simulink model "momentumBasedFlying"  (Simulink 10.3)
settings: Solver=FixedStepAuto  StartTime=0.0  StopTime=Config.simulationTime  FixedStep=Config.tStep  RelTol=1e-3
InitFcn:
  | cd(fileparts(which(bdroot)));
  | initMomentumBasedFlying;
StopFcn:
  | cd(fileparts(which(bdroot)));
  | stopMomentumBasedFlying;
undefined symbols (not defined in the file or in its folder): biasVectorConstraint_feet, Config, confVisualizer, ConstraintMatrix_feet, DiscIntNeverNeededParam, jets_config
libraries: WBToolboxLibrary x95, momentum_flight_control_sublib x2
(part 4 of 5)

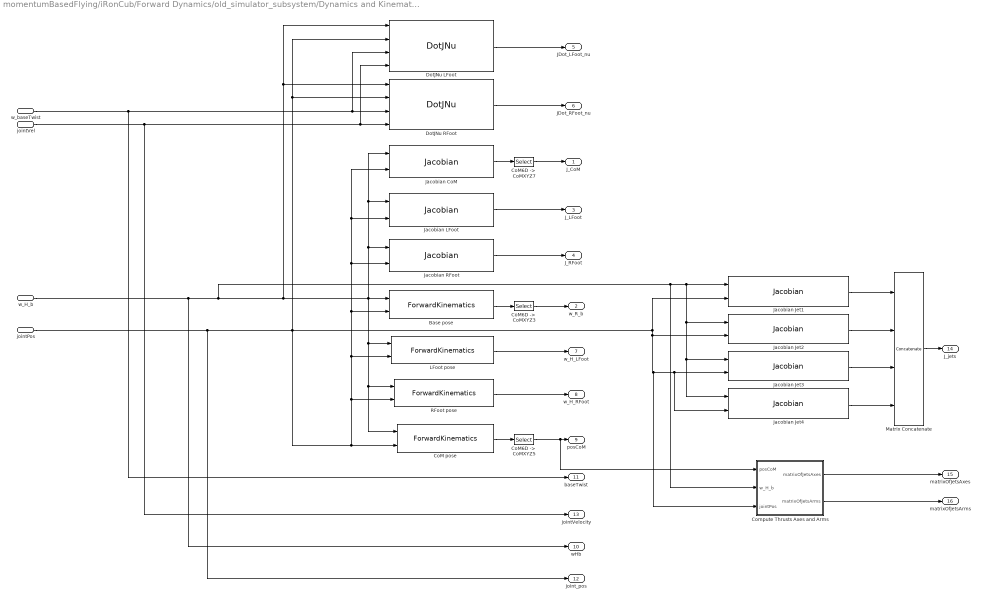
== system momentumBasedFlying/iRonCub/Forward Dynamics/old_simulator_subsystem/Dynamics and Kinematics/Kinematic Quantities ==
  w_H_b : Inport
  w_baseTwist : Inport  Port=2
  jointPos : Inport  Port=3
  jointVel : Inport  Port=4
  Base pose : WBToolboxLibrary/Model/Kinematics/ForwardKinematics  frameName=Frames.BASE_LINK
      settings: SourceProductName=WholeBodyToolbox
  CoM pose : WBToolboxLibrary/Model/Kinematics/ForwardKinematics  frameName=Frames.COM_FRAME
      settings: SourceProductName=WholeBodyToolbox
  "CoM6D ->  CoMXYZ3" : Selector  NumberOfDimensions=2  InputPortWidth=7  IndexOptions=Index vector (dialog),Index vector (dialog)  Indices=[1 2 3],[1 2 3]  OutputSizes=1,1
  "CoM6D ->  CoMXYZ5" : Selector  NumberOfDimensions=2  InputPortWidth=7  IndexOptions=Index vector (dialog),Index vector (dialog)  Indices=[1 2 3],[4]  OutputSizes=1,1
  "CoM6D ->  CoMXYZ7" : Selector  NumberOfDimensions=2  InputPortWidth=7  IndexOptions=Index vector (dialog),Index vector (dialog)  Indices=[1 2 3],[1:6+Config.N_DOF]  OutputSizes=1,1
  Compute Thrusts Axes and Arms : Subsystem
  DotJNu LFoot : WBToolboxLibrary/Model/Jacobians/DotJNu  frameName=Frames.LFOOT_FRAME
      settings: SourceProductName=WholeBodyToolbox
  DotJNu RFoot : WBToolboxLibrary/Model/Jacobians/DotJNu  frameName=Frames.RFOOT_FRAME
      settings: SourceProductName=WholeBodyToolbox
  Jacobian CoM : WBToolboxLibrary/Model/Jacobians/Jacobian  frameName=Frames.COM_FRAME
      settings: SourceProductName=WholeBodyToolbox
  Jacobian Jet1 : WBToolboxLibrary/Model/Jacobians/Jacobian  frameName=Frames.JET1_FRAME
      settings: SourceProductName=WholeBodyToolbox
  Jacobian Jet2 : WBToolboxLibrary/Model/Jacobians/Jacobian  frameName=Frames.JET2_FRAME
      settings: SourceProductName=WholeBodyToolbox
  Jacobian Jet3 : WBToolboxLibrary/Model/Jacobians/Jacobian  frameName=Frames.JET3_FRAME
      settings: SourceProductName=WholeBodyToolbox
  Jacobian Jet4 : WBToolboxLibrary/Model/Jacobians/Jacobian  frameName=Frames.JET4_FRAME
      settings: SourceProductName=WholeBodyToolbox
  Jacobian LFoot : WBToolboxLibrary/Model/Jacobians/Jacobian  frameName=Frames.LFOOT_FRAME
      settings: SourceProductName=WholeBodyToolbox
  Jacobian RFoot : WBToolboxLibrary/Model/Jacobians/Jacobian  frameName=Frames.RFOOT_FRAME
      settings: SourceProductName=WholeBodyToolbox
  LFoot pose : WBToolboxLibrary/Model/Kinematics/ForwardKinematics  frameName=Frames.LFOOT_FRAME
      settings: SourceProductName=WholeBodyToolbox
  Matrix Concatenate : Concatenate  NumInputs=4  Mode=Multidimensional array
  RFoot pose : WBToolboxLibrary/Model/Kinematics/ForwardKinematics  frameName=Frames.RFOOT_FRAME
      settings: SourceProductName=WholeBodyToolbox
  J_CoM : Outport  VectorParamsAs1DForOutWhenUnconnected=off
  w_R_b : Outport  Port=2  VectorParamsAs1DForOutWhenUnconnected=off
  J_LFoot : Outport  Port=3  VectorParamsAs1DForOutWhenUnconnected=off
  J_RFoot : Outport  Port=4  VectorParamsAs1DForOutWhenUnconnected=off
  JDot_LFoot_nu : Outport  Port=5  VectorParamsAs1DForOutWhenUnconnected=off
  JDot_RFoot_nu : Outport  Port=6  VectorParamsAs1DForOutWhenUnconnected=off
  w_H_LFoot : Outport  Port=7  VectorParamsAs1DForOutWhenUnconnected=off
  w_H_RFoot : Outport  Port=8  VectorParamsAs1DForOutWhenUnconnected=off
  posCoM : Outport  Port=9  VectorParamsAs1DForOutWhenUnconnected=off
  wHb : Outport  Port=10
  baseTwist : Outport  Port=11
  joint_pos : Outport  Port=12
  jointVelocity : Outport  Port=13
  J_jets : Outport  Port=14  VectorParamsAs1DForOutWhenUnconnected=off
  matrixOfJetsAxes : Outport  Port=15  VectorParamsAs1DForOutWhenUnconnected=off
  matrixOfJetsArms : Outport  Port=16  VectorParamsAs1DForOutWhenUnconnected=off
  wires:
  CoM pose/1 -> "CoM6D ->  CoMXYZ5"/1
  "CoM6D ->  CoMXYZ3"/1 -> w_R_b/1
  Jacobian CoM/1 -> "CoM6D ->  CoMXYZ7"/1
  Jacobian RFoot/1 -> J_RFoot/1
  Jacobian LFoot/1 -> J_LFoot/1
  DotJNu RFoot/1 -> JDot_RFoot_nu/1
  DotJNu LFoot/1 -> JDot_LFoot_nu/1
  jointVel/1 -> jointVelocity/1, DotJNu RFoot/4, DotJNu LFoot/4
  w_baseTwist/1 -> baseTwist/1, DotJNu LFoot/3, DotJNu RFoot/3
  RFoot pose/1 -> w_H_RFoot/1
  LFoot pose/1 -> w_H_LFoot/1
  Base pose/1 -> "CoM6D ->  CoMXYZ3"/1
  "CoM6D ->  CoMXYZ7"/1 -> J_CoM/1
  Compute Thrusts Axes and Arms/1(matrixOfJetsAxes) -> matrixOfJetsAxes/1
  Compute Thrusts Axes and Arms/2(matrixOfJetsArms) -> matrixOfJetsArms/1
  w_H_b/1 -> Compute Thrusts Axes and Arms/2(w_H_b), Jacobian Jet4/1, Jacobian Jet3/1, Jacobian Jet2/1, Jacobian Jet1/1, DotJNu LFoot/1, DotJNu RFoot/1, Jacobian LFoot/1, Jacobian CoM/1, Jacobian RFoot/1, CoM pose/1, RFoot pose/1, LFoot pose/1, Base pose/1, wHb/1
  Matrix Concatenate/1 -> J_jets/1
  Jacobian Jet3/1 -> Matrix Concatenate/3
  jointPos/1 -> Jacobian Jet4/2, Jacobian Jet3/2, Compute Thrusts Axes and Arms/3(jointPos), Jacobian Jet2/2, Jacobian Jet1/2, LFoot pose/2, Jacobian RFoot/2, Jacobian LFoot/2, Jacobian CoM/2, Base pose/2, RFoot pose/2, CoM pose/2, DotJNu RFoot/2, DotJNu LFoot/2, joint_pos/1
  Jacobian Jet4/1 -> Matrix Concatenate/4
  Jacobian Jet1/1 -> Matrix Concatenate/1
  Jacobian Jet2/1 -> Matrix Concatenate/2
  "CoM6D ->  CoMXYZ5"/1 -> Compute Thrusts Axes and Arms/1(posCoM), posCoM/1

== system momentumBasedFlying/FLYING CONTROLLER (CORE) V2.5/Dynamics and Kinematics/Dynamic Quantities/Momentum and CentroidalMomentum Matrix/CentroidalMomentum Matrix iCub 23/25 DoFs/CMM_base ==
  w_H_b : Inport
  jointPos : Inport  Port=2
  CentroidalMomentum{21..25,31} (6 alike) : WBToolboxLibrary/Model/Dynamics/CentroidalMomentum
      settings: SourceProductName=WholeBodyToolbox
  Constant : Constant  Value=[1,0,0,0,0,0]
  Constant1 : Constant  Value=[0,1,0,0,0,0]
  Constant2 : Constant  Value=zeros(Config.N_DOF,1)
  Constant3 : Constant  Value=[0,0,0,1,0,0]
  Constant37 : Constant  Value=[0,0,1,0,0,0]
  Constant4 : Constant  Value=[0,0,0,0,1,0]
  Constant6 : Constant  Value=[0,0,0,0,0,1]
  Matrix Concatenate : Concatenate  NumInputs=6  Mode=Multidimensional array  ConcatenateDimension=2
  CMM_base : Outport  VectorParamsAs1DForOutWhenUnconnected=off
  wires:
  w_H_b/1 -> CentroidalMomentum31/1, CentroidalMomentum25/1, CentroidalMomentum24/1, CentroidalMomentum23/1, CentroidalMomentum22/1, CentroidalMomentum21/1
  jointPos/1 -> CentroidalMomentum31/2, CentroidalMomentum25/2, CentroidalMomentum24/2, CentroidalMomentum23/2, CentroidalMomentum22/2, CentroidalMomentum21/2
  CentroidalMomentum25/1 -> Matrix Concatenate/5
  Matrix Concatenate/1 -> CMM_base/1
  CentroidalMomentum23/1 -> Matrix Concatenate/3
  CentroidalMomentum24/1 -> Matrix Concatenate/4
  CentroidalMomentum31/1 -> Matrix Concatenate/6
  Constant6/1 -> CentroidalMomentum31/3
  Constant/1 -> CentroidalMomentum21/3
  Constant1/1 -> CentroidalMomentum22/3
  Constant37/1 -> CentroidalMomentum23/3
  Constant2/1 -> CentroidalMomentum21/4, CentroidalMomentum31/4, CentroidalMomentum25/4, CentroidalMomentum24/4, CentroidalMomentum23/4, CentroidalMomentum22/4
  Constant4/1 -> CentroidalMomentum25/3
  Constant3/1 -> CentroidalMomentum24/3
  CentroidalMomentum22/1 -> Matrix Concatenate/2
  CentroidalMomentum21/1 -> Matrix Concatenate/1

== system momentumBasedFlying/FLYING CONTROLLER (CORE) V2.5/Dynamics and Kinematics/Dynamic Quantities/Momentum and CentroidalMomentum Matrix/CentroidalMomentum Matrix iCub 23/25 DoFs/CMM_joints ==
  w_H_b : Inport
  jointPos : Inport  Port=2
  SelMatrix : Inport  Port=3
  CMM Joints Group 1 : Subsystem
  CMM Joints Group 2 : Subsystem
  CMM Joints Group 3 : Subsystem
  CMM Joints Group 4 : Subsystem
  CMM Joints Group 5 : Subsystem
  Matrix Concatenate6 : Concatenate  NumInputs=4  Mode=Multidimensional array  ConcatenateDimension=2
  CMM_joints_from_1_to_20 : Outport  VectorParamsAs1DForOutWhenUnconnected=off
  CMM_group5_25DoFs : Outport  Port=2  VectorParamsAs1DForOutWhenUnconnected=off
  CMM_group5_23DoFs : Outport  Port=3  VectorParamsAs1DForOutWhenUnconnected=off
  wires:
  Matrix Concatenate6/1 -> CMM_joints_from_1_to_20/1
  w_H_b/1 -> CMM Joints Group 1/1(w_H_b), CMM Joints Group 2/1(w_H_b), CMM Joints Group 3/1(w_H_b), CMM Joints Group 4/1(w_H_b), CMM Joints Group 5/1(w_H_b)
  jointPos/1 -> CMM Joints Group 2/2(jointPos), CMM Joints Group 1/2(jointPos), CMM Joints Group 3/2(jointPos), CMM Joints Group 4/2(jointPos), CMM Joints Group 5/2(jointPos)
  SelMatrix/1 -> CMM Joints Group 3/3(SelMatrix), CMM Joints Group 2/3(SelMatrix), CMM Joints Group 1/3(SelMatrix), CMM Joints Group 4/3(SelMatrix), CMM Joints Group 5/3(SelMatrix)
  CMM Joints Group 1/1(CMM_group1) -> Matrix Concatenate6/1
  CMM Joints Group 2/1(CMM_group2) -> Matrix Concatenate6/2
  CMM Joints Group 3/1(CMM_group3) -> Matrix Concatenate6/3
  CMM Joints Group 4/1(CMM_group4) -> Matrix Concatenate6/4
  CMM Joints Group 5/1(CMM_group5_25DoFs) -> CMM_group5_25DoFs/1
  CMM Joints Group 5/2(CMM_group5_23DoFs) -> CMM_group5_23DoFs/1

== system momentumBasedFlying/FLYING CONTROLLER (CORE) V2.5/Dynamics and Kinematics/Dynamic Quantities/Momentum and CentroidalMomentum Matrix/CentroidalMomentum Matrix iCub 23/25 DoFs/Combine CMM ==
  CMM_base : Inport
  CMM_joints_1_20 : Inport  Port=2
  CMM_group5_25DoFs : Inport  Port=3
  CMM_group5_23DoFs : Inport  Port=4
  Matrix Concatenate1 : Concatenate  Mode=Multidimensional array  ConcatenateDimension=2
  Matrix Concatenate2 : Concatenate  Mode=Multidimensional array  ConcatenateDimension=2
  Matrix Concatenate6 : Concatenate  Mode=Multidimensional array  ConcatenateDimension=2
  CMM_25DoFs : Outport  VectorParamsAs1DForOutWhenUnconnected=off
  CMM_23DoFs : Outport  Port=2  VectorParamsAs1DForOutWhenUnconnected=off
  wires:
  Matrix Concatenate2/1 -> CMM_25DoFs/1
  Matrix Concatenate1/1 -> CMM_23DoFs/1
  CMM_group5_23DoFs/1 -> Matrix Concatenate1/2
  CMM_group5_25DoFs/1 -> Matrix Concatenate2/2
  Matrix Concatenate6/1 -> Matrix Concatenate2/1, Matrix Concatenate1/1
  CMM_base/1 -> Matrix Concatenate6/1
  CMM_joints_1_20/1 -> Matrix Concatenate6/2

== system momentumBasedFlying/FLYING CONTROLLER (CORE) V2.5/Flight Controller RAL-HUMANOIDS V3.1/Momentum Control for Flying/QP Solver and Integrate Contact Forces Derivative/Integrate the Contact Forces Derivative/deadZone ==
  u : Inport
  Constant : Constant  Value=Config.sat.deadZoneThreshold
  Deadzone Function : MATLAB Function  TreatAsAtomicUnit=on
  u_cut : Outport  VectorParamsAs1DForOutWhenUnconnected=off
  wires:
  Constant/1 -> Deadzone Function/2(thr)
  u/1 -> Deadzone Function/1(u)
  Deadzone Function/1(y) -> u_cut/1

== system momentumBasedFlying/FLYING CONTROLLER (CORE) V2.5/Flight Controller RAL-HUMANOIDS V3.1/Momentum Control for Flying/QP Solver and Integrate Contact Forces Derivative/QP momentumControl/QP momentumControl - balancing ==
  H : Inport
  g : Inport  Port=2
  ub : Inport  Port=3
  lb : Inport  Port=4
  Enable : EnablePort
  Constant : Constant  Value=eye(Config.N_DOF + 12 + 4)
  MatchSignalSizes : WBToolboxLibrary/Utilities/MatchSignalSizes
      settings: SourceProductName=WholeBodyToolbox
  QP : WBToolboxLibrary/Utilities/QP  lbA=on  ubA=on  lb=off  ub=off  computeObjVal=off  stopIfFails=off
      settings: SourceProductName=WholeBodyToolbox
  QPStatus_balancing : Outport  VectorParamsAs1DForOutWhenUnconnected=off
  QPOutput_balancing : Outport  Port=2  VectorParamsAs1DForOutWhenUnconnected=off
  wires:
  ub/1 -> QP/5
  QP/1 -> MatchSignalSizes/2
  MatchSignalSizes/1 -> QPOutput_balancing/1
  QP/2 -> QPStatus_balancing/1
  H/1 -> QP/1
  g/1 -> MatchSignalSizes/1, QP/2
  lb/1 -> QP/4
  Constant/1 -> QP/3

== system momentumBasedFlying/FLYING CONTROLLER (CORE) V2.5/Flight Controller RAL-HUMANOIDS V3.1/Momentum Control for Flying/QP Solver and Integrate Contact Forces Derivative/QP momentumControl/QP momentumControl - flight ==
  H : Inport
  g : Inport  Port=2
  ub : Inport  Port=3
  lb : Inport  Port=4
  Enable : EnablePort
  Constant : Constant  Value=eye(Config.N_DOF + 4)
  MatchSignalSizes : WBToolboxLibrary/Utilities/MatchSignalSizes
      settings: SourceProductName=WholeBodyToolbox
  QP flight-momentumControl : WBToolboxLibrary/Utilities/QP  lbA=on  ubA=on  lb=off  ub=off  computeObjVal=off  stopIfFails=off
      settings: SourceProductName=WholeBodyToolbox
  QPStatus_flight : Outport  VectorParamsAs1DForOutWhenUnconnected=off
  QPOutput_flight : Outport  Port=2  VectorParamsAs1DForOutWhenUnconnected=off
  wires:
  ub/1 -> QP flight-momentumControl/5
  g/1 -> MatchSignalSizes/1, QP flight-momentumControl/2
  H/1 -> QP flight-momentumControl/1
  QP flight-momentumControl/1 -> MatchSignalSizes/2
  MatchSignalSizes/1 -> QPOutput_flight/1
  lb/1 -> QP flight-momentumControl/4
  QP flight-momentumControl/2 -> QPStatus_flight/1
  Constant/1 -> QP flight-momentumControl/3

== system momentumBasedFlying/FLYING CONTROLLER (CORE) V2.5/Flight Controller RAL-HUMANOIDS V3.1/Momentum Control for Flying/QP Solver and Integrate Contact Forces Derivative/QP momentumControl/Select QP momentumControl Output ==
  QPStatus_balancing : Inport
  QPOutput_balancing : Inport  Port=2
  feetContactIsActive : Inport  Port=3
  QPStatus_flight : Inport  Port=4
  QPOutput_flight : Inport  Port=5
  Constant : Constant  Value=zeros(12,1)
  Demux : Demux  Outputs=[4;12;Config.N_DOF]
  Demux1 : Demux  Outputs=[4;Config.N_DOF]
  Switch{,1..3} (4 alike) : Switch  Criteria=u2 > Threshold
  jetsIntensitiesDot_star : Outport  VectorParamsAs1DForOutWhenUnconnected=off
  contactForcesDot_star : Outport  Port=2  VectorParamsAs1DForOutWhenUnconnected=off
  jointVel_star : Outport  Port=3  VectorParamsAs1DForOutWhenUnconnected=off
  exitFlagQP_momentumControl : Outport  Port=4  VectorParamsAs1DForOutWhenUnconnected=off
  wires:
  Demux1/2 -> Switch3/3
  Demux/3 -> Switch3/1
  Constant/1 -> Switch2/3
  Demux/2 -> Switch2/1
  Demux1/1 -> Switch1/3
  Demux/1 -> Switch1/1
  QPOutput_flight/1 -> Demux1/1
  QPOutput_balancing/1 -> Demux/1
  Switch/1 -> exitFlagQP_momentumControl/1
  QPStatus_flight/1 -> Switch/3
  QPStatus_balancing/1 -> Switch/1
  feetContactIsActive/1 -> Switch/2, Switch1/2, Switch2/2, Switch3/2
  Switch3/1 -> jointVel_star/1
  Switch1/1 -> jetsIntensitiesDot_star/1
  Switch2/1 -> contactForcesDot_star/1

== system momentumBasedFlying/FLYING CONTROLLER (CORE) V2.5/Flying Controller v2.5/Momentum Control for Flying/QP Solver and Integrate Contact Forces Derivative/Integrate the Contact Forces Derivative/deadZone ==
  u : Inport
  Constant : Constant  Value=Config.sat.deadZoneThreshold
  Deadzone Function : MATLAB Function  TreatAsAtomicUnit=on
  u_cut : Outport  VectorParamsAs1DForOutWhenUnconnected=off
  wires:
  Deadzone Function/1(y) -> u_cut/1
  u/1 -> Deadzone Function/1(u)
  Constant/1 -> Deadzone Function/2(thr)

== system momentumBasedFlying/FLYING CONTROLLER (CORE) V2.5/Flying State Machine/Compute Gains And References/Smooth CoM and Base References/Smooth Reference Orientations/Rotational PID Controller ==
  w_R_b_des : Inport
  gainSmoothingBaseRot : Inport  Port=2
  Compute Rotation Matrix Derivative : MATLAB Function  TreatAsAtomicUnit=on
  Discrete-Time Integrator2 : DiscreteIntegrator  InitialConditionSource=external  InitialCondition=zeros(3,1)  SampleTime=Config.tStep  ICPrevOutput=DiscIntNeverNeededParam  ICPrevScaledInput=DiscIntNeverNeededParam
  "holder " : WBToolboxLibrary/Utilities/holder 
      settings: SourceProductName=WholeBodyToolbox
  w_R_b_des_smooth : Outport  VectorParamsAs1DForOutWhenUnconnected=off
  body_omega_b_des_smooth : Outport  Port=2  VectorParamsAs1DForOutWhenUnconnected=off
  wires:
  "holder "/1 -> Discrete-Time Integrator2/2
  Compute Rotation Matrix Derivative/2(RDot) -> Discrete-Time Integrator2/1
  Discrete-Time Integrator2/1 -> w_R_b_des_smooth/1, Compute Rotation Matrix Derivative/3(w_R_b)
  w_R_b_des/1 -> "holder "/1, Compute Rotation Matrix Derivative/2(w_R_b_des)
  Compute Rotation Matrix Derivative/1(b_omega_b) -> body_omega_b_des_smooth/1
  gainSmoothingBaseRot/1 -> Compute Rotation Matrix Derivative/1(gainSmoothingBaseRot)

== system momentumBasedFlying/iRonCub/Forward Dynamics/old_simulator_subsystem/Dynamics and Kinematics/Kinematic Quantities/Compute Thrusts Axes and Arms ==
  posCoM : Inport
  w_H_b : Inport  Port=2
  jointPos : Inport  Port=3
  Pose Jet 1 : WBToolboxLibrary/Model/Kinematics/ForwardKinematics  frameName=Frames.JET1_FRAME
      settings: SourceProductName=WholeBodyToolbox
  Pose Jet 2 : WBToolboxLibrary/Model/Kinematics/ForwardKinematics  frameName=Frames.JET2_FRAME
      settings: SourceProductName=WholeBodyToolbox
  Pose Jet 3 : WBToolboxLibrary/Model/Kinematics/ForwardKinematics  frameName=Frames.JET3_FRAME
      settings: SourceProductName=WholeBodyToolbox
  Pose Jet 4 : WBToolboxLibrary/Model/Kinematics/ForwardKinematics  frameName=Frames.JET4_FRAME
      settings: SourceProductName=WholeBodyToolbox
  Thrust Axes and Arms : MATLAB Function  TreatAsAtomicUnit=on
  matrixOfJetsAxes : Outport  VectorParamsAs1DForOutWhenUnconnected=off
  matrixOfJetsArms : Outport  Port=2  VectorParamsAs1DForOutWhenUnconnected=off
  wires:
  Pose Jet 2/1 -> Thrust Axes and Arms/2(w_H_J2)
  jointPos/1 -> Pose Jet 1/2, Pose Jet 2/2, Pose Jet 3/2, Pose Jet 4/2
  Pose Jet 1/1 -> Thrust Axes and Arms/1(w_H_J1)
  Pose Jet 3/1 -> Thrust Axes and Arms/3(w_H_J3)
  Pose Jet 4/1 -> Thrust Axes and Arms/4(w_H_J4)
  Thrust Axes and Arms/1(matrixOfJetsAxes) -> matrixOfJetsAxes/1
  Thrust Axes and Arms/2(matrixOfJetsArms) -> matrixOfJetsArms/1
  w_H_b/1 -> Pose Jet 4/1, Pose Jet 3/1, Pose Jet 2/1, Pose Jet 1/1
  posCoM/1 -> Thrust Axes and Arms/5(posCoM)

== system momentumBasedFlying/FLYING CONTROLLER (CORE) V2.5/Dynamics and Kinematics/Dynamic Quantities/Momentum and CentroidalMomentum Matrix/CentroidalMomentum Matrix iCub 23/25 DoFs/CMM_joints/CMM Joints Group 1 ==
  w_H_b : Inport
  jointPos : Inport  Port=2
  SelMatrix : Inport  Port=3
  CentroidalMomentum{1..4,16} (5 alike) : WBToolboxLibrary/Model/Dynamics/CentroidalMomentum
      settings: SourceProductName=WholeBodyToolbox
  Constant : Constant  Value=zeros(6,1)
  Constant1 : Constant
  MATLAB Function : MATLAB Function  TreatAsAtomicUnit=on
  Matrix Concatenate6 : Concatenate  NumInputs=5  Mode=Multidimensional array  ConcatenateDimension=2
  CMM_group1 : Outport  VectorParamsAs1DForOutWhenUnconnected=off
  wires:
  Constant/1 -> CentroidalMomentum4/3, CentroidalMomentum3/3, CentroidalMomentum1/3, CentroidalMomentum16/3, CentroidalMomentum2/3
  CentroidalMomentum2/1 -> Matrix Concatenate6/3
  CentroidalMomentum1/1 -> Matrix Concatenate6/2
  CentroidalMomentum3/1 -> Matrix Concatenate6/4
  CentroidalMomentum16/1 -> Matrix Concatenate6/1
  w_H_b/1 -> CentroidalMomentum1/1, CentroidalMomentum2/1, CentroidalMomentum3/1, CentroidalMomentum4/1, CentroidalMomentum16/1
  CentroidalMomentum4/1 -> Matrix Concatenate6/5
  Matrix Concatenate6/1 -> CMM_group1/1
  MATLAB Function/1(v1) -> CentroidalMomentum16/4
  MATLAB Function/2(v2) -> CentroidalMomentum1/4
  MATLAB Function/3(v3) -> CentroidalMomentum2/4
  MATLAB Function/4(v4) -> CentroidalMomentum3/4
  MATLAB Function/5(v5) -> CentroidalMomentum4/4
  SelMatrix/1 -> MATLAB Function/1(SelMatrix)
  Constant1/1 -> MATLAB Function/2(groupNumber)
  jointPos/1 -> MATLAB Function/3(jointPos), CentroidalMomentum4/2, CentroidalMomentum3/2, CentroidalMomentum2/2, CentroidalMomentum16/2, CentroidalMomentum1/2

== system momentumBasedFlying/FLYING CONTROLLER (CORE) V2.5/Dynamics and Kinematics/Dynamic Quantities/Momentum and CentroidalMomentum Matrix/CentroidalMomentum Matrix iCub 23/25 DoFs/CMM_joints/CMM Joints Group 2 ==
  w_H_b : Inport
  jointPos : Inport  Port=2
  SelMatrix : Inport  Port=3
  CentroidalMomentum{1..4,16} (5 alike) : WBToolboxLibrary/Model/Dynamics/CentroidalMomentum
      settings: SourceProductName=WholeBodyToolbox
  Constant : Constant  Value=zeros(6,1)
  Constant1 : Constant  Value=2
  MATLAB Function : MATLAB Function  TreatAsAtomicUnit=on
  Matrix Concatenate6 : Concatenate  NumInputs=5  Mode=Multidimensional array  ConcatenateDimension=2
  CMM_group2 : Outport  VectorParamsAs1DForOutWhenUnconnected=off
  wires:
  Constant/1 -> CentroidalMomentum4/3, CentroidalMomentum3/3, CentroidalMomentum1/3, CentroidalMomentum16/3, CentroidalMomentum2/3
  CentroidalMomentum2/1 -> Matrix Concatenate6/3
  CentroidalMomentum1/1 -> Matrix Concatenate6/2
  CentroidalMomentum3/1 -> Matrix Concatenate6/4
  CentroidalMomentum16/1 -> Matrix Concatenate6/1
  w_H_b/1 -> CentroidalMomentum1/1, CentroidalMomentum2/1, CentroidalMomentum3/1, CentroidalMomentum4/1, CentroidalMomentum16/1
  CentroidalMomentum4/1 -> Matrix Concatenate6/5
  Matrix Concatenate6/1 -> CMM_group2/1
  MATLAB Function/1(v1) -> CentroidalMomentum16/4
  MATLAB Function/2(v2) -> CentroidalMomentum1/4
  MATLAB Function/3(v3) -> CentroidalMomentum2/4
  MATLAB Function/4(v4) -> CentroidalMomentum3/4
  MATLAB Function/5(v5) -> CentroidalMomentum4/4
  SelMatrix/1 -> MATLAB Function/1(SelMatrix)
  Constant1/1 -> MATLAB Function/2(groupNumber)
  jointPos/1 -> MATLAB Function/3(jointPos), CentroidalMomentum4/2, CentroidalMomentum3/2, CentroidalMomentum2/2, CentroidalMomentum16/2, CentroidalMomentum1/2

== system momentumBasedFlying/FLYING CONTROLLER (CORE) V2.5/Dynamics and Kinematics/Dynamic Quantities/Momentum and CentroidalMomentum Matrix/CentroidalMomentum Matrix iCub 23/25 DoFs/CMM_joints/CMM Joints Group 3 ==
  w_H_b : Inport
  jointPos : Inport  Port=2
  SelMatrix : Inport  Port=3
  CentroidalMomentum{1..4,16} (5 alike) : WBToolboxLibrary/Model/Dynamics/CentroidalMomentum
      settings: SourceProductName=WholeBodyToolbox
  Constant : Constant  Value=zeros(6,1)
  Constant1 : Constant  Value=3
  MATLAB Function : MATLAB Function  TreatAsAtomicUnit=on
  Matrix Concatenate6 : Concatenate  NumInputs=5  Mode=Multidimensional array  ConcatenateDimension=2
  CMM_group3 : Outport  VectorParamsAs1DForOutWhenUnconnected=off
  wires:
  Constant/1 -> CentroidalMomentum4/3, CentroidalMomentum3/3, CentroidalMomentum1/3, CentroidalMomentum16/3, CentroidalMomentum2/3
  CentroidalMomentum2/1 -> Matrix Concatenate6/3
  CentroidalMomentum1/1 -> Matrix Concatenate6/2
  CentroidalMomentum3/1 -> Matrix Concatenate6/4
  CentroidalMomentum16/1 -> Matrix Concatenate6/1
  w_H_b/1 -> CentroidalMomentum1/1, CentroidalMomentum2/1, CentroidalMomentum3/1, CentroidalMomentum4/1, CentroidalMomentum16/1
  CentroidalMomentum4/1 -> Matrix Concatenate6/5
  Matrix Concatenate6/1 -> CMM_group3/1
  MATLAB Function/1(v1) -> CentroidalMomentum16/4
  MATLAB Function/2(v2) -> CentroidalMomentum1/4
  MATLAB Function/3(v3) -> CentroidalMomentum2/4
  MATLAB Function/4(v4) -> CentroidalMomentum3/4
  MATLAB Function/5(v5) -> CentroidalMomentum4/4
  SelMatrix/1 -> MATLAB Function/1(SelMatrix)
  Constant1/1 -> MATLAB Function/2(groupNumber)
  jointPos/1 -> MATLAB Function/3(jointPos), CentroidalMomentum4/2, CentroidalMomentum3/2, CentroidalMomentum2/2, CentroidalMomentum16/2, CentroidalMomentum1/2

== system momentumBasedFlying/FLYING CONTROLLER (CORE) V2.5/Dynamics and Kinematics/Dynamic Quantities/Momentum and CentroidalMomentum Matrix/CentroidalMomentum Matrix iCub 23/25 DoFs/CMM_joints/CMM Joints Group 4 ==
  w_H_b : Inport
  jointPos : Inport  Port=2
  SelMatrix : Inport  Port=3
  CentroidalMomentum{1..4,16} (5 alike) : WBToolboxLibrary/Model/Dynamics/CentroidalMomentum
      settings: SourceProductName=WholeBodyToolbox
  Constant : Constant  Value=zeros(6,1)
  Constant1 : Constant  Value=4
  MATLAB Function : MATLAB Function  TreatAsAtomicUnit=on
  Matrix Concatenate6 : Concatenate  NumInputs=5  Mode=Multidimensional array  ConcatenateDimension=2
  CMM_group4 : Outport  VectorParamsAs1DForOutWhenUnconnected=off
  wires:
  Constant/1 -> CentroidalMomentum4/3, CentroidalMomentum3/3, CentroidalMomentum1/3, CentroidalMomentum16/3, CentroidalMomentum2/3
  CentroidalMomentum2/1 -> Matrix Concatenate6/3
  CentroidalMomentum1/1 -> Matrix Concatenate6/2
  CentroidalMomentum3/1 -> Matrix Concatenate6/4
  CentroidalMomentum16/1 -> Matrix Concatenate6/1
  w_H_b/1 -> CentroidalMomentum1/1, CentroidalMomentum2/1, CentroidalMomentum3/1, CentroidalMomentum4/1, CentroidalMomentum16/1
  CentroidalMomentum4/1 -> Matrix Concatenate6/5
  Matrix Concatenate6/1 -> CMM_group4/1
  MATLAB Function/1(v1) -> CentroidalMomentum16/4
  MATLAB Function/2(v2) -> CentroidalMomentum1/4
  MATLAB Function/3(v3) -> CentroidalMomentum2/4
  MATLAB Function/4(v4) -> CentroidalMomentum3/4
  MATLAB Function/5(v5) -> CentroidalMomentum4/4
  SelMatrix/1 -> MATLAB Function/1(SelMatrix)
  Constant1/1 -> MATLAB Function/2(groupNumber)
  jointPos/1 -> MATLAB Function/3(jointPos), CentroidalMomentum4/2, CentroidalMomentum3/2, CentroidalMomentum2/2, CentroidalMomentum16/2, CentroidalMomentum1/2

== system momentumBasedFlying/FLYING CONTROLLER (CORE) V2.5/Dynamics and Kinematics/Dynamic Quantities/Momentum and CentroidalMomentum Matrix/CentroidalMomentum Matrix iCub 23/25 DoFs/CMM_joints/CMM Joints Group 5 ==
  w_H_b : Inport
  jointPos : Inport  Port=2
  SelMatrix : Inport  Port=3
  CentroidalMomentum{1..4,16} (5 alike) : WBToolboxLibrary/Model/Dynamics/CentroidalMomentum
      settings: SourceProductName=WholeBodyToolbox
  Constant : Constant  Value=zeros(6,1)
  Constant1 : Constant  Value=5
  MATLAB Function : MATLAB Function  TreatAsAtomicUnit=on
  Matrix Concatenate1 : Concatenate  Mode=Multidimensional array  ConcatenateDimension=2
  Matrix Concatenate2 : Concatenate  Mode=Multidimensional array  ConcatenateDimension=2
  Matrix Concatenate6 : Concatenate  NumInputs=3  Mode=Multidimensional array  ConcatenateDimension=2
  CMM_group5_25DoFs : Outport  VectorParamsAs1DForOutWhenUnconnected=off
  CMM_group5_23DoFs : Outport  Port=2  VectorParamsAs1DForOutWhenUnconnected=off
  wires:
  Constant/1 -> CentroidalMomentum4/3, CentroidalMomentum3/3, CentroidalMomentum1/3, CentroidalMomentum16/3, CentroidalMomentum2/3
  CentroidalMomentum2/1 -> Matrix Concatenate6/3
  CentroidalMomentum1/1 -> Matrix Concatenate6/2
  jointPos/1 -> CentroidalMomentum4/2, MATLAB Function/3(jointPos), CentroidalMomentum3/2, CentroidalMomentum2/2, CentroidalMomentum16/2, CentroidalMomentum1/2
  CentroidalMomentum16/1 -> Matrix Concatenate6/1
  w_H_b/1 -> CentroidalMomentum1/1, CentroidalMomentum2/1, CentroidalMomentum3/1, CentroidalMomentum4/1, CentroidalMomentum16/1
  MATLAB Function/1(v1) -> CentroidalMomentum16/4
  MATLAB Function/2(v2) -> CentroidalMomentum1/4
  MATLAB Function/3(v3) -> CentroidalMomentum2/4
  MATLAB Function/4(v4) -> CentroidalMomentum3/4
  MATLAB Function/5(v5) -> CentroidalMomentum4/4
  SelMatrix/1 -> MATLAB Function/1(SelMatrix)
  Constant1/1 -> MATLAB Function/2(groupNumber)
  Matrix Concatenate6/1 -> CMM_group5_23DoFs/1, Matrix Concatenate2/1
  CentroidalMomentum4/1 -> Matrix Concatenate1/2
  CentroidalMomentum3/1 -> Matrix Concatenate1/1
  Matrix Concatenate1/1 -> Matrix Concatenate2/2
  Matrix Concatenate2/1 -> CMM_group5_25DoFs/1

== matlab function Visualizer/Task and Base Frame Kinematics/MATLAB Function1 ==
  data: RPY_Corr output double; rollPitchYaw input double
function RPY_Corr = correctYawAngleFCN(rollPitchYaw)

    RPY_Corr = correctYawAngle(rollPitchYaw);

end

== matlab function iRonCub/Forward Dynamics/old_simulator_subsystem/MATLAB Function1 ==
  data: base_linear_velocity output double; mass_matrix input double; bias_forces input double; joints_torque input double; generalized_ext_wrench input double; base_velocity input double; joints_velocity input double; JLeft_frameJac input double; JRight_frameJac input double; JDot_nu_LFOOT input double; JDot_nu_RFOOT input double; H_LFOOT input double; H_RFOOT input double; Config parameter double; omega_b output double; joints_velocity output double; dot_v_b output double; dot_omega_b output double; joint_acceleration output double; contact_detected output double; wrench_left_foot output double; wrench_right_foot output double
function [base_linear_velocity, omega_b, joints_velocity, dot_v_b, dot_omega_b, joint_acceleration, ...
    contact_detected, wrench_left_foot, wrench_right_foot] = ...
    forward_and_contact_dynamics(mass_matrix, bias_forces, joints_torque, generalized_ext_wrench, ...
    base_velocity, joints_velocity, JLeft_frameJac, JRight_frameJac, JDot_nu_LFOOT, JDot_nu_RFOOT, H_LFOOT, H_RFOOT, Config)

[base_linear_velocity, omega_b, joints_velocity, dot_v_b, dot_omega_b, joint_acceleration, ...
    contact_detected, wrench_left_foot, wrench_right_foot] = ...
    forward_and_contact_dynamics(mass_matrix, bias_forces, joints_torque, generalized_ext_wrench, ...
    base_velocity, joints_velocity, JLeft_frameJac, JRight_frameJac, JDot_nu_LFOOT, JDot_nu_RFOOT, H_LFOOT, H_RFOOT, Config);
end

== matlab function Visualizer/Task and Base Frame Kinematics/MATLAB Function3 ==
  data: RPY_Corr output double; rollPitchYaw input double
function RPY_Corr = correctYawAngleFCN(rollPitchYaw)

    RPY_Corr = correctYawAngle(rollPitchYaw);

end

== matlab function Visualizer/Task and Base Frame Kinematics/Get RPY from rotation matrix  ==
  data: w_R_b input double; rollPitchYaw output double
function rollPitchYaw = rollPitchYawFromRotationFCN(w_R_b)

rollPitchYaw = wbc.rollPitchYawFromRotation(w_R_b);

end

== matlab function FLYING CONTROLLER (CORE) V2.5/Dynamics and Kinematics/Dynamic Quantities/Compute Centroidal Inertia/Compute Centroidal Inertia ==
  data: M input double; w_I_c output double; posCoM input double; posBase input double
function w_I_c = getCentrInertiaFCN(M, posCoM, posBase)

    w_I_c = getCentrInertia(M, posCoM, posBase);
end

== matlab function Visualizer/Task and Base Frame Kinematics/Get RPY from rotation matrix ==
  data: w_R_b input double; rollPitchYaw output double
function rollPitchYaw = rollPitchYawFromRotationFCN(w_R_b)

rollPitchYaw = wbc.rollPitchYawFromRotation(w_R_b);

end

== matlab function Visualizer/Task and Base Frame Kinematics/Get RPY error norm ==
  data: rot_err input double; rotErr_norm output double
function rotErr_norm = normFCN(rot_err)

rotErr_norm = norm(rot_err);

end

== matlab function FLYING CONTROLLER (CORE) V2.5/Dynamics and Kinematics/Dynamic Quantities/Momentum and CentroidalMomentum Matrix/CentroidalMomentum Matrix iCub 23//25 DoFs/Select CMM 23 or 25 ==
  data: CMM_25 input double; N_DOF input double; CMM output double; CMM_23 input double
function CMM = selectCMM_23_25_FCN(CMM_25, N_DOF, CMM_23)

    CMM = CMM_25;
    
    if N_DOF < 25
        
        % dynamic sizing of CMM not allowed
        CMM = [CMM_23, zeros(size(CMM,1),2)];
    end
end

== matlab function FLYING CONTROLLER (CORE) V2.5/Flying State Machine/Take Off//Landing State Detector/MATLAB Function ==
  data: wrench_l input double; feetContactIsActive output double; wrench_r input double; Config parameter double; robotIsLanded output double; oneFootIsInContact output double
function [feetContactIsActive, robotIsLanded, oneFootIsInContact] = feetContactActivationFCN(wrench_l, wrench_r, Config)

    [feetContactIsActive, robotIsLanded, oneFootIsInContact] = feetContactActivation(wrench_l, wrench_r, Config);
end

== matlab function Visualizer/Task and Base Frame Kinematics/MATLAB Function2 ==
  data: RPY_Corr output double; rollPitchYaw input double
function RPY_Corr = correctYawAngleFCN(rollPitchYaw)

    RPY_Corr = correctYawAngle(rollPitchYaw);

end

== matlab function FLYING CONTROLLER (CORE) V2.5/Flying Controller v2.5/Joint Torque Control for Flying/Torque Derivative Saturation/Saturate Torque Derivative ==
  data: u input double; uSat output double; u_0 input double; tStep input double; uDotMax input double
function uSat = saturateInputDerivativeFCN(u, u_0, tStep, uDotMax)

    uSat = wbc.saturateInputDerivative(u, u_0, tStep, uDotMax);
end

== matlab function JoyStick Commands/Replace Joystick with Native GUI ==
  data: gui_input input double; joyButtons output double; joyAxes output double
function [joyButtons,joyAxes] = fromGuiToJoystickFCN(gui_input)

    [joyButtons,joyAxes] = fromGuiToJoystick(gui_input);
end

== matlab function FLYING CONTROLLER (CORE) V2.5/Get System State/Change Contact Forces Representation/Change Contact Forces Representation ==
  data: contactForces_WBD input double; mixed_f_l_sole output double; w_R_l_sole input double; w_R_r_sole input double; mixed_f_r_sole output double
function [mixed_f_l_sole, mixed_f_r_sole] = fromBodyFrameToMixed_contactForcesFCN(contactForces_WBD, w_R_l_sole, w_R_r_sole)

    [mixed_f_l_sole, mixed_f_r_sole] = fromBodyFrameToMixed_contactForces(contactForces_WBD, w_R_l_sole, w_R_r_sole);
end

== matlab function FLYING CONTROLLER (CORE) V2.5/Flying State Machine/Compute Gains And References/Compute Gains/Diagonalize ==
  data: k input double; K output double
function K = diagonalMatrixFromVectorFCN(k)

    K = wbc.diagonalMatrixFromVector(k);
end

== matlab function FLYING CONTROLLER (CORE) V2.5/Flying State Machine/Compute Gains And References/Compute Gains/Diagonalize1 ==
  data: k input double; K output double
function K = diagonalMatrixFromVectorFCN(k)

    K = wbc.diagonalMatrixFromVector(k);
end

== matlab function FLYING CONTROLLER (CORE) V2.5/Flying State Machine/Compute Gains And References/Compute Gains/Diagonalize2 ==
  data: k input double; K output double
function K = diagonalMatrixFromVectorFCN(k)

    K = wbc.diagonalMatrixFromVector(k);
end

== matlab function FLYING CONTROLLER (CORE) V2.5/Flying Controller v2.5/Momentum Control for Flying/Momentum Control/Flying Controller Momentum FCN  ==
  data: jointPos input double; w_baseTwist input double; jetsIntensities input double; J_jets input double; J_CoM input double; J_LFoot input double; J_RFoot input double; posCoM input double; w_R_b input double; w_H_LFoot input double; w_H_RFoot input double; matrixOfJetsAxes input double; matrixOfJetsArms input double; w_I_c input double; L input double; M input double; CMM input double; pos_vel_acc_jerk_CoM_des input double; rot_vel_acc_jerk_base_des input double size=[3,6]; jointPos_des input double; KP_momentum input double; KD_momentum input double; KP_postural input double; feetContactIsActive input double; decreaseMaxFootVerticalForce input double; increaseMinFootVerticalForce input double; robotIsLanded input double; HessianMatrixQP output double; gVectorQP output double; lowerBoundQP output double; upperBoundQP output double; L_des output double size=[6,1]; LDot_estimated output double size=[6,1]; verifyAngMomAndInertia output double; contactForces_hat input double; Config parameter double
function [HessianMatrixQP, gVectorQP, lowerBoundQP, upperBoundQP, L_des, LDot_estimated, verifyAngMomAndInertia] = ...
             flyingMomentumControlFCN(jointPos, w_baseTwist, jetsIntensities, J_jets, J_CoM, J_LFoot, J_RFoot, posCoM, w_R_b, w_H_LFoot, ...
                                      w_H_RFoot, matrixOfJetsAxes, matrixOfJetsArms, w_I_c, L, M, CMM, pos_vel_acc_jerk_CoM_des, ....
                                      rot_vel_acc_jerk_base_des, jointPos_des, KP_momentum, KD_momentum, KP_postural, feetContactIsActive, ...
                                      decreaseMaxFootVerticalForce, increaseMinFootVerticalForce, robotIsLanded, contactForces_hat, Config)
                               
    [HessianMatrixQP, gVectorQP, lowerBoundQP, upperBoundQP, L_des, LDot_estimated , verifyAngMomAndInertia] = ...
        flyingMomentumControl(jointPos, w_baseTwist, jetsIntensities, J_jets, J_CoM, J_LFoot, J_RFoot, posCoM, w_R_b, w_H_LFoot, ...
                              w_H_RFoot, matrixOfJetsAxes, matrixOfJetsArms, w_I_c, L, M, CMM, pos_vel_acc_jerk_CoM_des, ....
                              rot_vel_acc_jerk_base_des, jointPos_des, KP_momentum, KD_momentum, KP_postural, feetContactIsActive, ...
                               decreaseMaxFootVerticalForce, increaseMinFootVerticalForce, robotIsLanded, contactForces_hat, Config);
end

== matlab function FLYING CONTROLLER (CORE) V2.5/Flying Controller v2.5/Joint Torque Control for Flying/torqueControlFCN ==
  data: M input double; h input double; J_jets input double; J_LFoot input double; J_RFoot input double; JDot_LFoot_nu input double; JDot_RFoot_nu input double; w_H_LFoot input double; w_H_RFoot input double; matrixOfJetsAxes input double; ConstraintsMatrix_feet input double; biasVectorConstraint_feet input double; jetsIntensities input double; stateVel input double; jointVel_star input double; contactForces_star input double; KI_torqueControl input double; KP_torqueControl input double; feetContactIsActive input double; activateEqConstrTorqueControl input double; robotIsLanded input double; jointPos_err input double; Hessian output double; Config parameter double; gradient output double; ConstraintMatrix_inequality output double; biasVectorConstraint_inequality output double; jointVel_err output double
function [Hessian, gradient, ConstraintMatrix_inequality, biasVectorConstraint_inequality, jointVel_err] =  ... 
             flyingTorqueControlFCN(M, h, J_jets, J_LFoot, J_RFoot, JDot_LFoot_nu, JDot_RFoot_nu, w_H_LFoot, w_H_RFoot, matrixOfJetsAxes, ...
                                    ConstraintsMatrix_feet, biasVectorConstraint_feet, jetsIntensities, stateVel, jointVel_star, contactForces_star, ...
                                    KI_torqueControl, KP_torqueControl, feetContactIsActive, activateEqConstrTorqueControl, robotIsLanded, jointPos_err, Config)
                                      
    [Hessian, gradient, ConstraintMatrix_inequality, biasVectorConstraint_inequality, jointVel_err] =  ... 
        flyingTorqueControl(M, h, J_jets, J_LFoot, J_RFoot, JDot_LFoot_nu, JDot_RFoot_nu, w_H_LFoot, w_H_RFoot, matrixOfJetsAxes, ...
                            ConstraintsMatrix_feet, biasVectorConstraint_feet, jetsIntensities, stateVel, jointVel_star, contactForces_star, ...
                            KI_torqueControl, KP_torqueControl, feetContactIsActive, activateEqConstrTorqueControl, robotIsLanded, jointPos_err, Config);           
end

== matlab function FLYING CONTROLLER (CORE) V2.5/Flying State Machine/Compute Gains And References/Compute Gains/Diagonalize3 ==
  data: k input double; K output double
function K = diagonalMatrixFromVectorFCN(k)

    K = wbc.diagonalMatrixFromVector(k);
end

== matlab function FLYING CONTROLLER (CORE) V2.5/Dynamics and Kinematics/Kinematic Quantities/Compute Thrusts Axes and Arms/Thrust Axes and Arms ==
  data: w_H_J1 input double; matrixOfJetsAxes output double; w_H_J2 input double; w_H_J3 input double; w_H_J4 input double; posCoM input double; matrixOfJetsArms output double; Config parameter double
function [matrixOfJetsAxes, matrixOfJetsArms] = computeJetsAxesAndArmsFCN(w_H_J1, w_H_J2, w_H_J3, w_H_J4, posCoM, Config)

    [matrixOfJetsAxes, matrixOfJetsArms] = computeJetsAxesAndArms(w_H_J1, w_H_J2, w_H_J3, w_H_J4, posCoM, Config);
end

== matlab function FLYING CONTROLLER (CORE) V2.5/Flying State Machine/Compute Gains And References/Compute Gains/Diagonalize4 ==
  data: k input double; K output double
function K = diagonalMatrixFromVectorFCN(k)

    K = wbc.diagonalMatrixFromVector(k);
end

== matlab function MATLAB Function ==
  data: t input double; v_wind output double
function v_wind= generate_windFCN(t)

v_wind=generate_wind(t);
end

== matlab function FLYING CONTROLLER (CORE) V2.5/Flying Controller v2.5/Momentum Control for Flying/QP Solver and Integrate Contact Forces Derivative/Integrate the Contact Forces Derivative/deadZone/Deadzone Function ==
  data: u input double; y output double; thr input double
function y = deadZoneFCN(u, thr)

    y = wbc.deadZone(u, thr);
end

== matlab function FLYING CONTROLLER (CORE) V2.5/Flying State Machine/Take Off//Landing State Detector/Vertical Forces Control ==
  data: joyButtons input double; decreaseMaxFootVerticalForce output double; increaseMinFootVerticalForce output double; activateEqConstrTorqueControl output double
function [decreaseMaxFootVerticalForce, increaseMinFootVerticalForce, activateEqConstrTorqueControl] = verticalForcesControlFCN(joyButtons)

    [decreaseMaxFootVerticalForce, increaseMinFootVerticalForce, activateEqConstrTorqueControl] = verticalForcesControl(joyButtons);
end

== matlab function FLYING CONTROLLER (CORE) V2.5/Dynamics and Kinematics/Dynamic Quantities/Momentum and CentroidalMomentum Matrix/CentroidalMomentum Matrix iCub 23//25 DoFs/CMM_joints/CMM Joints Group 1/MATLAB Function ==
  data: SelMatrix input double; v1 output double; groupNumber input double; v2 output double; v3 output double; v4 output double; v5 output double; jointPos input double
function [v1,v2,v3,v4,v5] = selectFiveMatrixColumns(SelMatrix,groupNumber,jointPos)
        
    ndof = length(jointPos);
    
    v1   = SelMatrix((groupNumber-1)*5 + 1,1:ndof);
    v2   = SelMatrix((groupNumber-1)*5 + 2,1:ndof);
    v3   = SelMatrix((groupNumber-1)*5 + 3,1:ndof);
    v4   = SelMatrix((groupNumber-1)*5 + 4,1:ndof);
    v5   = SelMatrix((groupNumber-1)*5 + 5,1:ndof);
end

== matlab function FLYING CONTROLLER (CORE) V2.5/Dynamics and Kinematics/Dynamic Quantities/Momentum and CentroidalMomentum Matrix/CentroidalMomentum Matrix iCub 23//25 DoFs/CMM_joints/CMM Joints Group 2/MATLAB Function ==
  data: SelMatrix input double; v1 output double; groupNumber input double; v2 output double; v3 output double; v4 output double; v5 output double; jointPos input double
function [v1,v2,v3,v4,v5] = selectFiveMatrixColumns(SelMatrix,groupNumber,jointPos)
        
    ndof = length(jointPos);
    
    v1   = SelMatrix((groupNumber-1)*5 + 1,1:ndof);
    v2   = SelMatrix((groupNumber-1)*5 + 2,1:ndof);
    v3   = SelMatrix((groupNumber-1)*5 + 3,1:ndof);
    v4   = SelMatrix((groupNumber-1)*5 + 4,1:ndof);
    v5   = SelMatrix((groupNumber-1)*5 + 5,1:ndof);
end

== matlab function FLYING CONTROLLER (CORE) V2.5/Dynamics and Kinematics/Dynamic Quantities/Momentum and CentroidalMomentum Matrix/CentroidalMomentum Matrix iCub 23//25 DoFs/CMM_joints/CMM Joints Group 3/MATLAB Function ==
  data: SelMatrix input double; v1 output double; groupNumber input double; v2 output double; v3 output double; v4 output double; v5 output double; jointPos input double
function [v1,v2,v3,v4,v5] = selectFiveMatrixColumns(SelMatrix,groupNumber,jointPos)
        
    ndof = length(jointPos);
    
    v1   = SelMatrix((groupNumber-1)*5 + 1,1:ndof);
    v2   = SelMatrix((groupNumber-1)*5 + 2,1:ndof);
    v3   = SelMatrix((groupNumber-1)*5 + 3,1:ndof);
    v4   = SelMatrix((groupNumber-1)*5 + 4,1:ndof);
    v5   = SelMatrix((groupNumber-1)*5 + 5,1:ndof);
end

== matlab function FLYING CONTROLLER (CORE) V2.5/Dynamics and Kinematics/Dynamic Quantities/Momentum and CentroidalMomentum Matrix/CentroidalMomentum Matrix iCub 23//25 DoFs/CMM_joints/CMM Joints Group 4/MATLAB Function ==
  data: SelMatrix input double; v1 output double; groupNumber input double; v2 output double; v3 output double; v4 output double; v5 output double; jointPos input double
function [v1,v2,v3,v4,v5] = selectFiveMatrixColumns(SelMatrix,groupNumber,jointPos)
        
    ndof = length(jointPos);
    
    v1   = SelMatrix((groupNumber-1)*5 + 1,1:ndof);
    v2   = SelMatrix((groupNumber-1)*5 + 2,1:ndof);
    v3   = SelMatrix((groupNumber-1)*5 + 3,1:ndof);
    v4   = SelMatrix((groupNumber-1)*5 + 4,1:ndof);
    v5   = SelMatrix((groupNumber-1)*5 + 5,1:ndof);
end

== matlab function FLYING CONTROLLER (CORE) V2.5/Dynamics and Kinematics/Dynamic Quantities/Momentum and CentroidalMomentum Matrix/CentroidalMomentum Matrix iCub 23//25 DoFs/CMM_joints/CMM Joints Group 5/MATLAB Function ==
  data: SelMatrix input double; v1 output double; groupNumber input double; v2 output double; v3 output double; v4 output double; v5 output double; jointPos input double
function [v1,v2,v3,v4,v5] = selectFiveMatrixColumns(SelMatrix,groupNumber,jointPos)
        
    ndof = length(jointPos);
    
    v1   = SelMatrix((groupNumber-1)*5 + 1,1:ndof);
    v2   = SelMatrix((groupNumber-1)*5 + 2,1:ndof);
    v3   = SelMatrix((groupNumber-1)*5 + 3,1:ndof);
    v4   = SelMatrix((groupNumber-1)*5 + 4,1:ndof);
    v5   = SelMatrix((groupNumber-1)*5 + 5,1:ndof);
end

== matlab function FLYING CONTROLLER (CORE) V2.5/Dynamics and Kinematics/Dynamic Quantities/Momentum and CentroidalMomentum Matrix/CentroidalMomentum Matrix iCub 23//25 DoFs/Selector Matrix ==
  data: ROBOT_DOF input double; SelMatrix output double; SelMatrix_0 input double
function SelMatrix = updateSelectorMatrix(ROBOT_DOF, SelMatrix_0)
    SelMatrix = blkdiag(SelMatrix_0, zeros(2));
end

== matlab function FLYING CONTROLLER (CORE) V2.5/Flying Controller v2.5/Momentum Control for Flying/QP Solver and Integrate Contact Forces Derivative/Integrate the Contact Forces Derivative/Select Integrator Initial Condition ==
  data: feetContactIsActive input double; contactForces input double; contactForces_0 output double
function contactForces_0 = selectInitContactForcesFCN(feetContactIsActive, contactForces)

    contactForces_0 = selectInitContactForces(feetContactIsActive, contactForces);
end

== matlab function FLYING CONTROLLER (CORE) V2.5/Flight Controller RAL-HUMANOIDS V3.1/Joint Torque Control for Flying/QP torqueControl/Process QP Inputs Torque Control ==
  data: HessianMatrixQP input double; H_balancing output double; gVectorQP input double; InequalityConstrMatrix input double; biasVectorInequalityConstr input double; g_balancing output double; ub_balancing output double; lb_balancing output double; Aeq_balancing output double; lbEq_balancing output double; ubEq_balancing output double; H_flight output double; g_flight output double; ub_flight output double; lb_flight output double; jointTorquesSaturation input double; Config parameter double
function [H_balancing,g_balancing,ub_balancing,lb_balancing,Aeq_balancing,lbEq_balancing,ubEq_balancing, ...
          H_flight,g_flight,ub_flight,lb_flight] = processQPinputTorqueControlFCN ...
                                                       (HessianMatrixQP,gVectorQP,InequalityConstrMatrix, ...
                                                        biasVectorInequalityConstr,jointTorquesSaturation,Config)   
   
[H_balancing,g_balancing,ub_balancing,lb_balancing,Aeq_balancing,lbEq_balancing,ubEq_balancing, ...
          H_flight,g_flight,ub_flight,lb_flight] = iRonCubLib.processQPinputTorqueControl ...
                                                       (HessianMatrixQP,gVectorQP,InequalityConstrMatrix, ...
                                                        biasVectorInequalityConstr,jointTorquesSaturation,Config);     
end

== matlab function FLYING CONTROLLER (CORE) V2.5/Flying State Machine/Compute Gains And References/Compute Gains/MATLAB Function ==
  data: KP_linear input double; KP_linear_t output double; KP2_linear input double; t input double
function KP_linear_t = gain_scheduling(KP_linear,KP2_linear,t)
% a=15/4;
% b=-15;
% c=15;
% if 5<=t && t<7
%     KP_linear_t=KP_linear+a*(t-5+(-b/2/a))^2+b*(t-5+(-b/2/a))+c;
% 
% else
%     KP_linear_t=KP_linear;
% end

if 6<=t && t<=8
    KP_linear_t=KP2_linear;
else
    KP_linear_t=KP_linear;
end




end

% elseif 8<=t && t<=10
%     KP_linear_t=KP_linear+a*(t-8)^2+b*(t-8)+c;

== matlab function FLYING CONTROLLER (CORE) V2.5/Flying Controller v2.5/Momentum Control for Flying/extendedKalmanFilter4jets/EKF_jet1/EKF  ==
  data: x input double; input input double; measurement input double; xDot output double; P input double; Config parameter double; Pdot output double
function [xDot, Pdot] = extendedKalmanFilterFNC(x, input, measurement, P, Config)

[xDot, Pdot] = extKalmanFilter(x, input, Config.jetC_P100, P, measurement, Config);

== matlab function FLYING CONTROLLER (CORE) V2.5/Flying Controller v2.5/Momentum Control for Flying/extendedKalmanFilter4jets/EKF_jet1/splitVector ==
  data: x input double; x1 output double; x2 output double
function [x1, x2] = fcn(x)
x1 = x(1);
x2 = x(2);

== matlab function iRonCub/Forward Dynamics/old_simulator_subsystem/Compute generalized external wrench and jet thrust/Compute generalized jet wrench/Jet Dynamics ==
  data: u input double; jetDerivativesOut output double; jetIntensities input double size=[4,1]; jetDerivatives input double size=[4,1]; Config parameter double; jetAccelerationOut output double
function [jetDerivativesOut, jetAccelerationOut] = fcn(u, jetIntensities, jetDerivatives, Config)
jetDerivativesOut = zeros(4,1);
jetAccelerationOut = zeros(4,1);
for i=1:4
    state = [jetIntensities(i), jetDerivatives(i)];
    x = jetModel.get_xDot(state, Config.jet.coeff(i,:), u(i));
    jetDerivativesOut(i) = x(1);
    jetAccelerationOut(i) = x(2);
end
end
